simulink model "Test"  (R2014a)
settings: Solver=FixedStepDiscrete  StartTime=0.0  StopTime=inf  FixedStep=SampleTime  RelTol=1e-3
libraries: visionstatistics x2, dspbuff3 x2, dspstat3 x2, dspmtrx3 x2
settings Model: Creator=georg  LastModifiedBy=georg

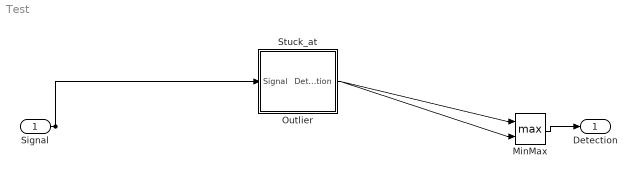
== system Test ==
  Signal : Inport
  MinMax : MinMax  Function=max  Inputs=2
  Outlier : Subsystem
  Stuck_at : Subsystem
  Detection : Outport
  wires:
  MinMax/1 -> Detection/1
  Signal/1 -> Outlier/1(Signal), Stuck_at/1(Signal)
  Outlier/1(Detection) -> MinMax/1
  Stuck_at/1(Detection) -> MinMax/2

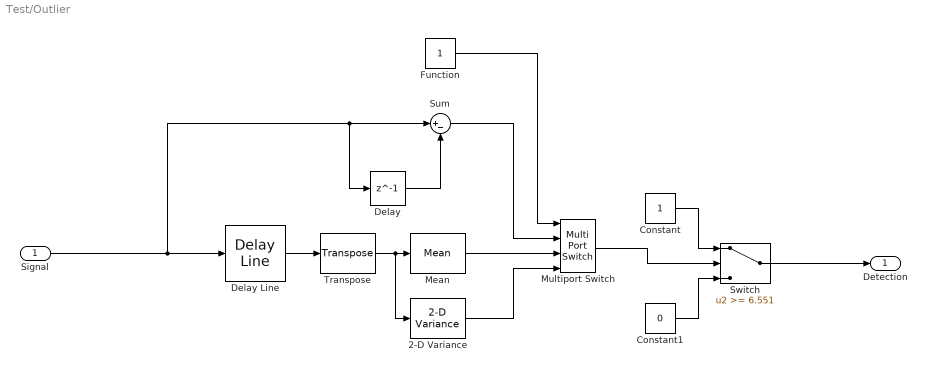
== system Test/Outlier ==
  Signal : Inport
  2-D Variance : visionstatistics/2-D Variance  run=off  reset_popup=None  directionMode=Entire input  dimension=1  treatSBRowAsCol=on  roiEnable=off  roiType=Rectangles  roiPortion=Entire ROI  roiOutput=Individual statistics for each ROI  roiFlag=off  prodOutputMode=Binary point scaling  prodOutputWordLength=32  prodOutputFracLength=0  roundingMode=Floor  overflowMode=off
  Constant : Constant
  Constant1 : Constant  Value=0
  Delay : Delay  DelayLength=1  InitialCondition=0
  Delay Line : dspbuff3/Delay Line  siz=1  ic=0  directfeed=off  enable_output=off  hold_output=off  TreatMby1Signals=One channel
  Function : Constant
  Mean : dspstat3/Mean  run=off  reset_popup=None  InputProcessing=Columns as channels (frame based)  directionMode=Each column  dimension=1  treatSBRowAsCol=on  roiEnable=off  roiType=Rectangles  roiPortion=Entire ROI  roiOutput=Individual statistics for each ROI  roiFlag=off  outputDataTypeStr=Inherit: Same as accumulator  outputLastDataTypeStr=Inherit: Same as accumulator  outputMin=[]  outputMax=[]  roundingMode=Floor  overflowMode=off
  Multiport Switch : MultiPortSwitch
  Sum : Sum  Inputs=|+-
  Switch : Switch  Threshold=6.551
  Transpose : dspmtrx3/Transpose  Hermitian=off  overflowFlag=off
  Detection : Outport
  wires:
  Sum/1 -> Multiport Switch/2
  Multiport Switch/1 -> Switch/2
  Delay/1 -> Sum/2
  Transpose/1 -> 2-D Variance/1, Mean/1
  Switch/1 -> Detection/1
  2-D Variance/1 -> Multiport Switch/4
  Signal/1 -> Delay Line/1, Sum/1, Delay/1
  Mean/1 -> Multiport Switch/3
  Constant1/1 -> Switch/3
  Constant/1 -> Switch/1
  Function/1 -> Multiport Switch/1
  Delay Line/1 -> Transpose/1

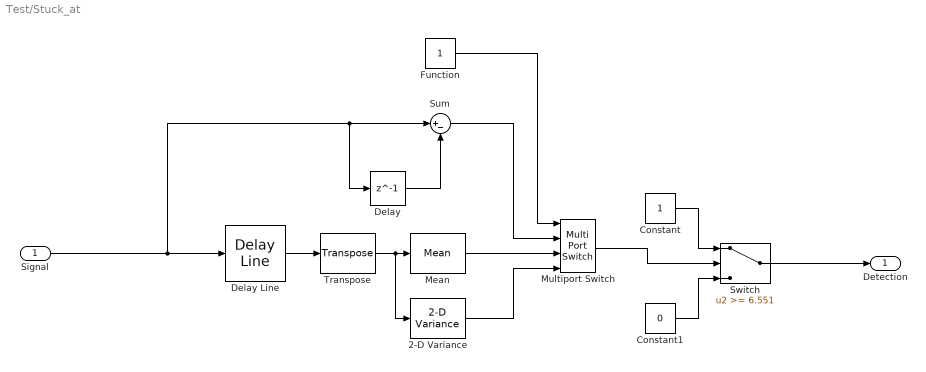
== system Test/Stuck_at ==
  Signal : Inport
  2-D Variance : visionstatistics/2-D Variance  run=off  reset_popup=None  directionMode=Entire input  dimension=1  treatSBRowAsCol=on  roiEnable=off  roiType=Rectangles  roiPortion=Entire ROI  roiOutput=Individual statistics for each ROI  roiFlag=off  prodOutputMode=Binary point scaling  prodOutputWordLength=32  prodOutputFracLength=0  roundingMode=Floor  overflowMode=off
  Constant : Constant
  Constant1 : Constant  Value=0
  Delay : Delay  DelayLength=1  InitialCondition=0
  Delay Line : dspbuff3/Delay Line  siz=1  ic=0  directfeed=off  enable_output=off  hold_output=off  TreatMby1Signals=One channel
  Function : Constant
  Mean : dspstat3/Mean  run=off  reset_popup=None  InputProcessing=Columns as channels (frame based)  directionMode=Each column  dimension=1  treatSBRowAsCol=on  roiEnable=off  roiType=Rectangles  roiPortion=Entire ROI  roiOutput=Individual statistics for each ROI  roiFlag=off  outputDataTypeStr=Inherit: Same as accumulator  outputLastDataTypeStr=Inherit: Same as accumulator  outputMin=[]  outputMax=[]  roundingMode=Floor  overflowMode=off
  Multiport Switch : MultiPortSwitch
  Sum : Sum  Inputs=|+-
  Switch : Switch  Threshold=6.551
  Transpose : dspmtrx3/Transpose  Hermitian=off  overflowFlag=off
  Detection : Outport
  wires:
  Sum/1 -> Multiport Switch/2
  Multiport Switch/1 -> Switch/2
  Delay/1 -> Sum/2
  Transpose/1 -> 2-D Variance/1, Mean/1
  Switch/1 -> Detection/1
  2-D Variance/1 -> Multiport Switch/4
  Signal/1 -> Delay Line/1, Sum/1, Delay/1
  Mean/1 -> Multiport Switch/3
  Constant1/1 -> Switch/3
  Constant/1 -> Switch/1
  Function/1 -> Multiport Switch/1
  Delay Line/1 -> Transpose/1
